simulink model "SwashPlateless_ESC"  (R2025b)
settings: Solver=VariableStepAuto  StartTime=0.0  StopTime=Stop_Time  FixedStep=1e-6  MaxStep=1e-6  RelTol=1e-4
values from neighbouring files (symbols this model uses):
  alpha_bp_rad = deg2rad(alpha_bp_deg)    [Check_alpha_sign.m]    (also in Swash.m)
  alpha_sign = alpha_sign_list(k)    [Check_alpha_sign.m]    (also in Swash.m = 1)
  B = 1.24e-5    (= 1.24e-05)    [Swash.m]
  Imax = 12    [Swash.m]
  J = 1.7e-5    (= 1.7e-05)    [Swash.m]
  Kac = Kic/Kpc    (= 237.676056338)    [Swash.m]
  Kh = 1    [Swash.m]
  Kic = Ra*Wcc    (= 127.23450247)    [Swash.m]
  Kpc = La*Wcc    (= 0.535327388172)    [Swash.m]
  KQ = T0/(W0^2)    (= 3.64756261112e-07)    [Swash.m]
  Kt = 60/(2*pi*KV)    (= 0.0203176523096)    [Swash.m]
  La = 2.84e-4    (= 0.000284)    [Swash.m]
  lambda_f = Kt/(1.5*p)    (= 0.00193501450568)    [Swash.m]
  p = 7    [Swash.m]
  phi_cmd = deg2rad(phi_cmd_deg)    [Check_alpha_sign.m]    (also in Swash.m = deg2rad(30); Sweep_param.m = deg2rad(phi_range_deg(j)))
  rpm_bp = [0 1000 2000 3000 4000 5000 6000]    [Swash.m]
  T0 = 0.10    (= 0.1)    [Swash.m]
  T1 = 0.01    [Check_alpha_sign.m]    (also in Swash.m; Sweep_param.m = T1_range(i))
  tau_h = 0.02    [Swash.m]
  theta_align = deg2rad(-3)    [Swash.m]
  Va_rated = Vdc    (= 22.2)    [Swash.m]
  Vdc = 22.2    [Swash.m]
  Wdisk = 2*pi*fdisk    (= 125.663706144)    [Swash.m]
  Wf = 2*pi*Ff    (= 6283.18530718)    [Swash.m]
undefined symbols (not defined in the file or in its folder): magnitude, plecs
libraries: slpidlib x2, plecslib_extras2 x2, simulink x1
settings Model: Creator=devil  LastModifiedBy=chyuj
settings DebuggingCC: MaxConsecutiveZCsMsg=warning

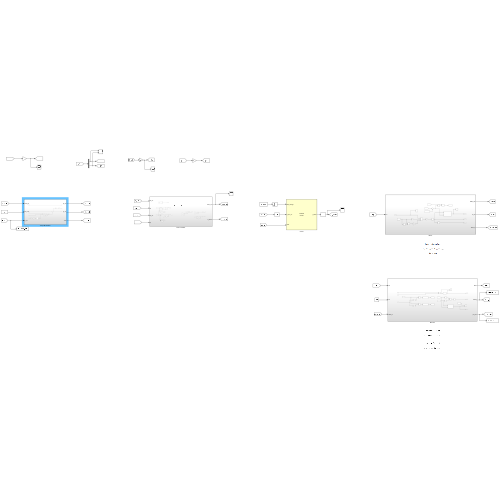
[thumbnail: Simulink's stored preview of the top-level diagram]
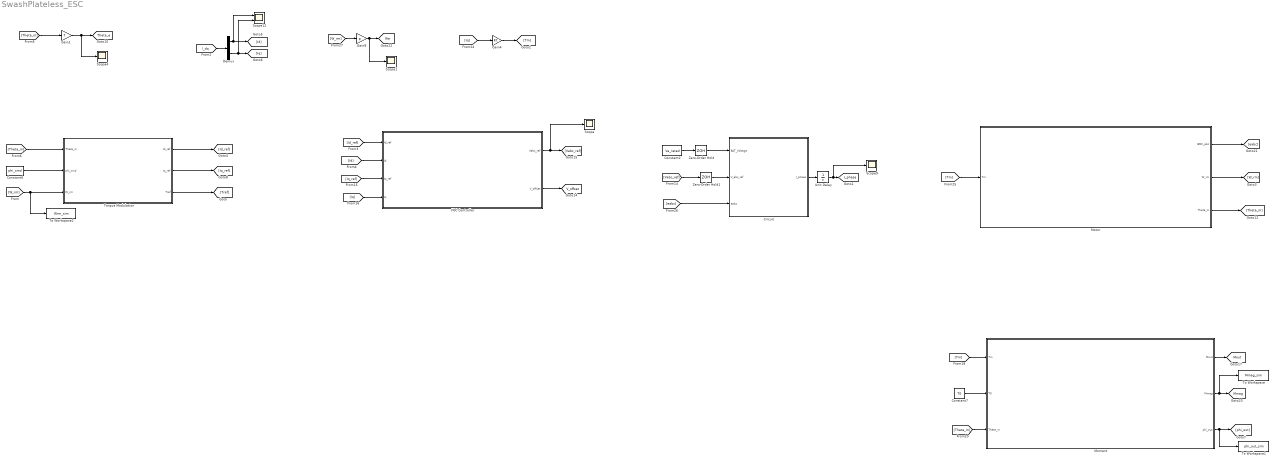
== system SwashPlateless_ESC ==
  Circuit : Subsystem  LoadFcn=plecs('sl', 200);  InitFcn=plecs('sl', 214);  StartFcn=plecs('sl', 208);  StopFcn=plecs('sl', 209);  mask(PlecsCircuit){PLECSData=<binary blob, 6192 chars, not shown>}
      mask prompts: PLECSData "PLECS Data (Do not delete or modify!)"
      mask init:
      | % PLACE CUSTOM INITIALIZATIONS ABOVE
      | % DO NOT REMOVE
      | plecs('sl', 215);
      | % DO NOT REMOVE
      settings: CopyFcn=plecs('sl', 203);  DeleteFcn=plecs('sl', 205);  UndoDeleteFcn=plecs('sl', 206);  PreSaveFcn=plecs('sl', 211);  PostSaveFcn=plecs('sl', 201);  NameChangeFcn=plecs('sl', 210);  DestroyFcn=plecs('sl', 207);  PreCopyFcn=plecs('sl', 216);  OpenFcn=plecs('sl', 202);  ErrorFcn=plerrorfcn
      mask Help: eval('plecs(''help'', ''qthelp:///creatingacircuit.html'')')
      mask Display: disp('PLECS\nCircuit')
  Constant2 : Constant  Value=Va_rated
  Constant6 : Constant  Value=phi_cmd
  Constant7 : Constant  Value=T0
  Demux : Demux  Outputs=2
  FOC Controller : Subsystem
  Gain1 : Gain  Gain=7
  Gain4 : Gain  Gain=Kt
  Gain8 : Gain  Gain=p
  Moment : Subsystem
  Motor : Subsystem
  Scope{,1,4,9} (4 alike) : Scope
      Scope settings: ActiveDisplayYMinimum=-4.6315212670934374  ActiveDisplayYMaximum=5.3776987823320246
      Scope1 settings: ActiveDisplayYMinimum=-1  ActiveDisplayYMaximum=1
      Scope4 settings: ActiveDisplayYMinimum=-1  ActiveDisplayYMaximum=1  DataLoggingVariableName=ScopeData2
      Scope9 settings: ActiveDisplayYMinimum=-6.552499916333363  ActiveDisplayYMaximum=6.5468585971785176  DataLoggingVariableName=ScopeData7
  Scope12 : Scope  NumInputPorts=2
      settings: ActiveDisplayYMinimum=-1.4248324543747475  ActiveDisplayYMaximum=7.121085765539088  DataLoggingVariableName=ScopeData10
  To Workspace : ToWorkspace  VariableName=Mmag_sim  SaveFormat=Timeseries  SampleTime=-1
  To Workspace1 : ToWorkspace  VariableName=phi_out_sim  SaveFormat=Timeseries  SampleTime=-1
  To Workspace2 : ToWorkspace  VariableName=Wrm_sim  SaveFormat=Timeseries  SampleTime=-1
  Torque Modulation : Subsystem
  Unit Delay : UnitDelay  SampleTime=-1  HasFrameUpgradeWarning=on
  Zero-Order Hold : ZeroOrderHold  SampleTime=-1
  Zero-Order Hold1 : ZeroOrderHold  SampleTime=-1
  tag scope: I_phase=global, Mmag=global, Mout=global, Theta_e=global, V_offset=global, We=global
  wires:
  [I_dq] -> Demux/1
  Demux/1 -> Scope12/1, [Id]
  Demux/2 -> Scope12/2, [Iq]
  [Vabc_ref] -> Zero-Order Hold1/1
  Constant2/1 -> Zero-Order Hold/1
  [Theta_m] -> Gain1/1
  Gain1/1 -> Scope4/1, [Theta_e]
  Circuit/1(I_phase) -> Unit Delay/1
  Unit Delay/1 -> Scope9/1, [I_phase]
  Zero-Order Hold/1 -> Circuit/1(BAT_Voltage)
  Zero-Order Hold1/1 -> Circuit/2(V_abc_ref)
  [Iq] -> Gain4/1
  Gain4/1 -> [Tm]
  [eabc] -> Circuit/3(eabc)
  [W_rm] -> Gain8/1
  Gain8/1 -> Scope1/1, [We]
  [Theta_m] -> Torque Modulation/1(Theta_m)
  Constant6/1 -> Torque Modulation/2(phi_cmd)
  Torque Modulation/2(Iq_ref) -> [Iq_ref]
  Torque Modulation/3(Tref) -> [Tref]
  FOC Controller/2(V_offset) -> [V_offset]
  FOC Controller/1(Vabc_ref) -> Scope/1, [Vabc_ref]
  [Id_ref] -> FOC Controller/1(Id_ref)
  [Id] -> FOC Controller/2(Id)
  [Iq_ref] -> FOC Controller/3(Iq_ref)
  [Iq] -> FOC Controller/4(Iq)
  [Tm] -> Moment/1(Tm)
  Constant7/1 -> Moment/2(T0)
  [Theta_m] -> Moment/3(Theta_m)
  Moment/1(Mout) -> [Mout]
  [Tm] -> Motor/1(Tm)
  Motor/1(BMF_abc) -> [eabc]
  Motor/2(W_rm) -> [W_rm]
  Motor/3(Theta_m) -> [Theta_m]
  Torque Modulation/1(Id_ref) -> [Id_ref]
  Moment/2(Mmag) -> To Workspace/1, [Mmag]
  Moment/3(phi_out) -> To Workspace1/1, [phi_out]
  [W_rm] -> To Workspace2/1, Torque Modulation/3(W_rm)

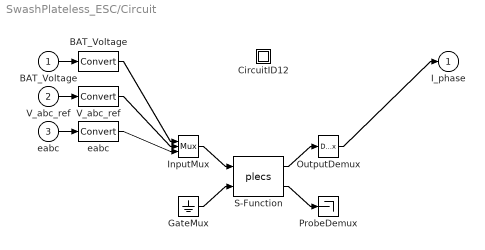
== system SwashPlateless_ESC/Circuit ==
  BAT_Voltage : Inport  PortDimensions=1
  V_abc_ref : Inport  Port=2  PortDimensions=3
  eabc : Inport  Port=3  PortDimensions=3
  " BAT_Voltage " : DataTypeConversion
  " CircuitID12 " : Subsystem
  " GateMux " : Ground
  " InputMux " : Mux  Inputs=[ 1 3 3 ]
  " OutputDemux " : Demux  Outputs=[ 3 ]
  " ProbeDemux " : Terminator
  " S-Function " : S-Function  FunctionName=plecs  SFunctionDeploymentMode=off  EnableBusSupport=off
  " V_abc_ref " : DataTypeConversion
  " eabc " : DataTypeConversion
  I_phase : Outport  PortDimensions=3
  wires:
  " InputMux "/1 -> " S-Function "/1
  " GateMux "/1 -> " S-Function "/2
  " S-Function "/1 -> " OutputDemux "/1
  " S-Function "/2 -> " ProbeDemux "/1
  BAT_Voltage/1 -> " BAT_Voltage "/1
  " BAT_Voltage "/1 -> " InputMux "/1
  V_abc_ref/1 -> " V_abc_ref "/1
  " V_abc_ref "/1 -> " InputMux "/2
  eabc/1 -> " eabc "/1
  " eabc "/1 -> " InputMux "/3
  " OutputDemux "/1 -> I_phase/1

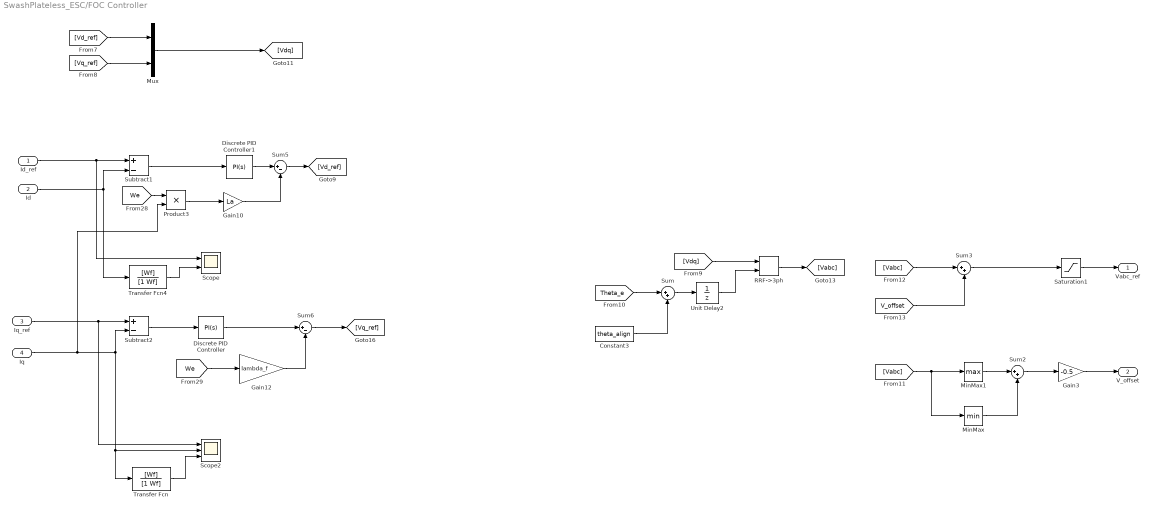
== system SwashPlateless_ESC/FOC Controller ==
  Id_ref : Inport
  Id : Inport  Port=2
  Iq_ref : Inport  Port=3
  Iq : Inport  Port=4
  Constant3 : Constant  Value=theta_align
  Discrete PID Controller : slpidlib/PID Controller  Controller=PI  Form=Parallel  TimeDomain=Continuous-time  UseExternalTs=off  SampleTime=-1  IntegratorMethod=Forward Euler  FilterMethod=Forward Euler  ControllerParametersSource=internal  P=Kpc  I=Kic  UseKiTs=off  D=0  UseExternalDerivativeSource=off  N=100  UseFilter=on  TunerSelectOption=Transfer Function Based (PID Tuner App)  InitialConditionSource=internal  InitialConditionForIntegrator=0  InitialConditionForFilter=0  DifferentiatorICPrevScaledInput=0  ExternalReset=none  TrackingMode=off  Kt=1  LimitOutput=on  SatLimitsSource=internal  UpperSaturationLimit=Vdc/sqrt(3)  LowerSaturationLimit=-Vdc/sqrt(3)  LinearizeAsGain=on  AntiWindupMode=back-calculation  Kb=Kac  LimitIntegrator=off  UpperIntegratorSaturationLimit=inf  LowerIntegratorSaturationLimit=-inf  POutMin=[]  POutMax=[]  IOutMin=[]  IOutMax=[]  DOutMin=[]  DOutMax=[]  NOutMin=[]  NOutMax=[]  SumOutMin=[]  SumOutMax=[]  SaturationOutMin=[]  SaturationOutMax=[]  PParamMin=[]  PParamMax=[]  IParamMin=[]  IParamMax=[]  DParamMin=[]  DParamMax=[]  NParamMin=[]  NParamMax=[]  KbParamMin=[]  KbParamMax=[]  KtParamMin=[]  KtParamMax=[]  KbOutMin=[]  KbOutMax=[]  KtOutMin=[]  KtOutMax=[]  IntegratorOutMin=[]  IntegratorOutMax=[]  FilterOutMin=[]  FilterOutMax=[]  SumI1OutMin=[]  SumI1OutMax=[]  SumI2OutMin=[]  SumI2OutMax=[]  SumI3OutMin=[]  SumI3OutMax=[]  SumI4OutMin=[]  SumI4OutMax=[]  SumDOutMin=[]  SumDOutMax=[]  DifferentiatorOutMin=[]  DifferentiatorOutMax=[]  FilterDiffOutCoefMin=[]  FilterDiffOutCoefMax=[]  ReciprocalOutMin=[]  ReciprocalOutMax=[]  SumDenOutMin=[]  SumDenOutMax=[]  SumNumOutMin=[]  SumNumOutMax=[]  DivideOutMin=[]  DivideOutMax=[]  UdiffTsProdOutMin=[]  UdiffTsProdOutMax=[]  NTsProdOutMin=[]  NTsProdOutMax=[]  UintegralTsProdOutMin=[]  UintegralTsProdOutMax=[]  UngainTsProdOutMin=[]  UngainTsProdOutMax=[]  ClampingZeroOutDataTypeStr=Inherit: Inherit via back propagation  ClampingZeroOutMin=[]  ClampingZeroOutMax=[]  FilterDenConstantOutDataTypeStr=Inherit: Inherit via back propagation  FilterDenConstantOutMin=[]  FilterDenConstantOutMax=[]  PCopyOutDataTypeStr=Inherit: Inherit via back propagation  PCopyOutMin=[]  PCopyOutMax=[]  NCopyOutDataTypeStr=Inherit: Inherit via back propagation  NCopyOutMin=[]  NCopyOutMax=[]  IntegratorContinuousStateAttributes=''  IntegratorStateMustResolveToSignalObject=off  IntegratorRTWStateStorageClass=Auto  FilterContinuousStateAttributes=''  FilterStateMustResolveToSignalObject=off  FilterRTWStateStorageClass=Auto  ParallelPVariant=InternalParameters  IdealPVariant=Disabled  IVariant=InternalParameters  DVariant=Disabled  IntegratorVariant=Continuous  SatVariant=Enabled  AWVariant=BackCalculation  PCopyVariant=Disabled  TRVariant=Disabled  FdbkBlocksVariant=Forward  IdealPFdbkVariant=Disabled  SatFdbkVariant=Disabled  DerivativeFilterVariant=Disabled  NVariant=Disabled  NCopyVariant=Disabled_SignalSpec  FilterICVariant=Disabled  IntegratorICVariant=InternalICs  ExternalResetVariant=Disabled  TRSumVariant=Passthrough  SumFdbkVariant=Disabled  SumVariant=Sum_PI  TsampFilterVariant=InternalTs  TsampNgainVariant=Passthrough  TsampIntegralVariant=Disabled_SignalSpec  ExternalSaturationOutDataTypeStr=Inherit: Same as second input  DerivativeSourceVariant=Disabled  PreIntVariant=InternalPreInt
      settings: LibrarySourceBlock=simulink/Discrete/Discrete PID Controller
  Discrete PID Controller1 : slpidlib/PID Controller  Controller=PI  Form=Parallel  TimeDomain=Continuous-time  UseExternalTs=off  SampleTime=-1  IntegratorMethod=Forward Euler  FilterMethod=Forward Euler  ControllerParametersSource=internal  P=Kpc  I=Kic  UseKiTs=off  D=0  UseExternalDerivativeSource=off  N=100  UseFilter=on  TunerSelectOption=Transfer Function Based (PID Tuner App)  InitialConditionSource=internal  InitialConditionForIntegrator=0  InitialConditionForFilter=0  DifferentiatorICPrevScaledInput=0  ExternalReset=none  TrackingMode=off  Kt=1  LimitOutput=on  SatLimitsSource=internal  UpperSaturationLimit=Vdc/sqrt(3)  LowerSaturationLimit=-Vdc/sqrt(3)  LinearizeAsGain=on  AntiWindupMode=back-calculation  Kb=Kac  LimitIntegrator=off  UpperIntegratorSaturationLimit=inf  LowerIntegratorSaturationLimit=-inf  POutMin=[]  POutMax=[]  IOutMin=[]  IOutMax=[]  DOutMin=[]  DOutMax=[]  NOutMin=[]  NOutMax=[]  SumOutMin=[]  SumOutMax=[]  SaturationOutMin=[]  SaturationOutMax=[]  PParamMin=[]  PParamMax=[]  IParamMin=[]  IParamMax=[]  DParamMin=[]  DParamMax=[]  NParamMin=[]  NParamMax=[]  KbParamMin=[]  KbParamMax=[]  KtParamMin=[]  KtParamMax=[]  KbOutMin=[]  KbOutMax=[]  KtOutMin=[]  KtOutMax=[]  IntegratorOutMin=[]  IntegratorOutMax=[]  FilterOutMin=[]  FilterOutMax=[]  SumI1OutMin=[]  SumI1OutMax=[]  SumI2OutMin=[]  SumI2OutMax=[]  SumI3OutMin=[]  SumI3OutMax=[]  SumI4OutMin=[]  SumI4OutMax=[]  SumDOutMin=[]  SumDOutMax=[]  DifferentiatorOutMin=[]  DifferentiatorOutMax=[]  FilterDiffOutCoefMin=[]  FilterDiffOutCoefMax=[]  ReciprocalOutMin=[]  ReciprocalOutMax=[]  SumDenOutMin=[]  SumDenOutMax=[]  SumNumOutMin=[]  SumNumOutMax=[]  DivideOutMin=[]  DivideOutMax=[]  UdiffTsProdOutMin=[]  UdiffTsProdOutMax=[]  NTsProdOutMin=[]  NTsProdOutMax=[]  UintegralTsProdOutMin=[]  UintegralTsProdOutMax=[]  UngainTsProdOutMin=[]  UngainTsProdOutMax=[]  ClampingZeroOutDataTypeStr=Inherit: Inherit via back propagation  ClampingZeroOutMin=[]  ClampingZeroOutMax=[]  FilterDenConstantOutDataTypeStr=Inherit: Inherit via back propagation  FilterDenConstantOutMin=[]  FilterDenConstantOutMax=[]  PCopyOutDataTypeStr=Inherit: Inherit via back propagation  PCopyOutMin=[]  PCopyOutMax=[]  NCopyOutDataTypeStr=Inherit: Inherit via back propagation  NCopyOutMin=[]  NCopyOutMax=[]  IntegratorContinuousStateAttributes=''  IntegratorStateMustResolveToSignalObject=off  IntegratorRTWStateStorageClass=Auto  FilterContinuousStateAttributes=''  FilterStateMustResolveToSignalObject=off  FilterRTWStateStorageClass=Auto  ParallelPVariant=InternalParameters  IdealPVariant=Disabled  IVariant=InternalParameters  DVariant=Disabled  IntegratorVariant=Continuous  SatVariant=Enabled  AWVariant=BackCalculation  PCopyVariant=Disabled  TRVariant=Disabled  FdbkBlocksVariant=Forward  IdealPFdbkVariant=Disabled  SatFdbkVariant=Disabled  DerivativeFilterVariant=Disabled  NVariant=Disabled  NCopyVariant=Disabled_SignalSpec  FilterICVariant=Disabled  IntegratorICVariant=InternalICs  ExternalResetVariant=Disabled  TRSumVariant=Passthrough  SumFdbkVariant=Disabled  SumVariant=Sum_PI  TsampFilterVariant=InternalTs  TsampNgainVariant=Passthrough  TsampIntegralVariant=Disabled_SignalSpec  ExternalSaturationOutDataTypeStr=Inherit: Same as second input  DerivativeSourceVariant=Disabled  PreIntVariant=InternalPreInt
      settings: LibrarySourceBlock=simulink/Discrete/Discrete PID Controller
  Gain10 : Gain  Gain=La
  Gain12 : Gain  Gain=lambda_f
  Gain3 : Gain  Gain=-0.5
  MinMax : MinMax
  MinMax1 : MinMax  Function=max
  Mux : Mux  Inputs=2
  Product3 : Product
  RRF->3ph : plecslib_extras2/Transformations/RRF->3ph
      settings: SourceProductName=PLECS Extras
  Saturation1 : Saturate  UpperLimit=0.49*Vdc  LowerLimit=-0.49*Vdc
  Scope : Scope  NumInputPorts=2
      settings: ActiveDisplayYMinimum=-2.7389602608191588  ActiveDisplayYMaximum=3.7222976897141629
  Scope2 : Scope  NumInputPorts=3
      settings: ActiveDisplayYMinimum=4.9459750721392517  ActiveDisplayYMaximum=5.2413041360162866  DataLoggingVariableName=ScopeData2
  Subtract1 : Sum  Inputs=+-
  Subtract2 : Sum  Inputs=+-
  Sum : Sum  Inputs=|++
  Sum2 : Sum  Inputs=|++
  Sum3 : Sum  Inputs=|++
  Sum5 : Sum  Inputs=|+-
  Sum6 : Sum  Inputs=|+-
  Transfer Fcn : TransferFcn  Numerator=[Wf]  Denominator=[1 Wf]
  Transfer Fcn4 : TransferFcn  Numerator=[Wf]  Denominator=[1 Wf]
  Unit Delay2 : UnitDelay  SampleTime=-1  HasFrameUpgradeWarning=on
  Vabc_ref : Outport
  V_offset : Outport  Port=2
  wires:
  Sum5/1 -> [Vd_ref]
  [Vdq] -> RRF->3ph/1
  Id_ref/1 -> Scope/1, Subtract1/1
  Iq/1 -> Product3/2, Subtract2/2, Transfer Fcn/1, Scope2/2
  Id/1 -> Transfer Fcn4/1, Subtract1/2
  Sum6/1 -> [Vq_ref]
  Iq_ref/1 -> Scope2/1, Subtract2/1
  Discrete PID Controller1/1 -> Sum5/1
  MinMax/1 -> Sum2/2
  Subtract2/1 -> Discrete PID Controller/1
  Constant3/1 -> Sum/2
  Mux/1 -> [Vdq]
  [Theta_e] -> Sum/1
  [Vabc] -> MinMax/1, MinMax1/1
  Gain10/1 -> Sum5/2
  [V_offset] -> Sum3/2
  Subtract1/1 -> Discrete PID Controller1/1
  [Vd_ref] -> Mux/1
  Transfer Fcn/1 -> Scope2/3
  Discrete PID Controller/1 -> Sum6/1
  Gain12/1 -> Sum6/2
  Sum2/1 -> Gain3/1
  Transfer Fcn4/1 -> Scope/2
  [We] -> Product3/1
  Unit Delay2/1 -> RRF->3ph/2
  Sum/1 -> Unit Delay2/1
  [Vq_ref] -> Mux/2
  [Vabc] -> Sum3/1
  Sum3/1 -> Saturation1/1
  [We] -> Gain12/1
  Gain3/1 -> V_offset/1
  Product3/1 -> Gain10/1
  MinMax1/1 -> Sum2/1
  RRF->3ph/1 -> [Vabc]
  Saturation1/1 -> Vabc_ref/1

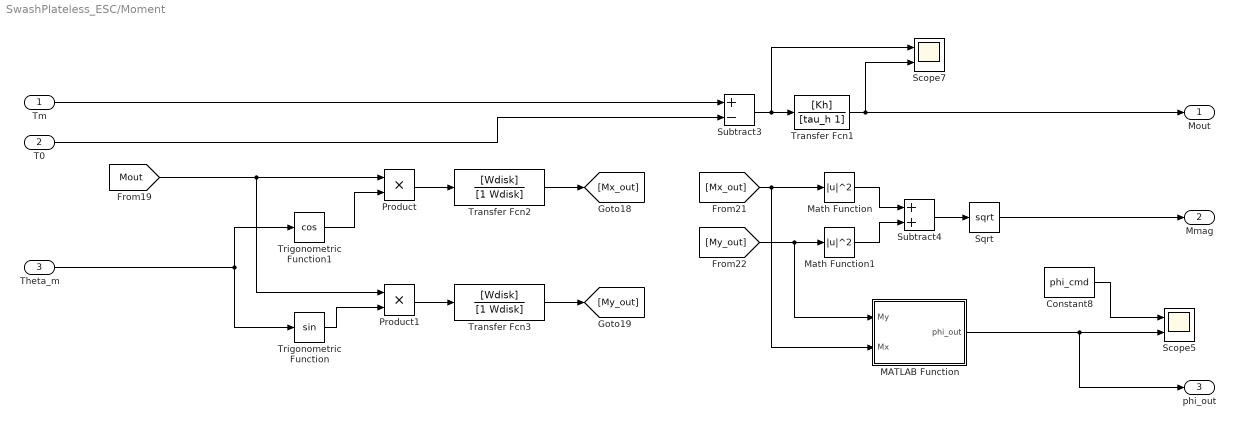
== system SwashPlateless_ESC/Moment ==
  Tm : Inport
  T0 : Inport  Port=2
  Theta_m : Inport  Port=3
  Constant8 : Constant  Value=phi_cmd
  MATLAB Function : MATLAB Function  TreatAsAtomicUnit=on
  Math Function : Math  Operator=magnitude^2
  Math Function1 : Math  Operator=magnitude^2
  Product : Product
  Product1 : Product
  Scope5 : Scope  NumInputPorts=2
      settings: ActiveDisplayYMinimum=-1  ActiveDisplayYMaximum=1  DataLoggingVariableName=ScopeData3
  Scope7 : Scope  NumInputPorts=2
      settings: ActiveDisplayYMinimum=-0.11471706424926205  ActiveDisplayYMaximum=0.032453578243358414  DataLoggingVariableName=ScopeData5
  Sqrt : Sqrt
  Subtract3 : Sum  Inputs=+-
  Subtract4 : Sum
  Transfer Fcn1 : TransferFcn  Numerator=[Kh]  Denominator=[tau_h 1]
  Transfer Fcn2 : TransferFcn  Numerator=[Wdisk]  Denominator=[1 Wdisk]
  Transfer Fcn3 : TransferFcn  Numerator=[Wdisk]  Denominator=[1 Wdisk]
  Trigonometric Function : Trigonometry
  Trigonometric Function1 : Trigonometry  Operator=cos
  Mout : Outport
  Mmag : Outport  Port=2
  phi_out : Outport  Port=3
  wires:
  Math Function1/1 -> Subtract4/2
  Theta_m/1 -> Trigonometric Function/1, Trigonometric Function1/1
  [Mx_out] -> MATLAB Function/2(Mx), Math Function/1
  Transfer Fcn2/1 -> [Mx_out]
  MATLAB Function/1(phi_out) -> phi_out/1, Scope5/2
  Product/1 -> Transfer Fcn2/1
  Constant8/1 -> Scope5/1
  Transfer Fcn1/1 -> Mout/1, Scope7/2
  Product1/1 -> Transfer Fcn3/1
  Subtract3/1 -> Scope7/1, Transfer Fcn1/1
  [My_out] -> MATLAB Function/1(My), Math Function1/1
  Transfer Fcn3/1 -> [My_out]
  [Mout] -> Product1/1, Product/1
  Trigonometric Function1/1 -> Product/2
  Subtract4/1 -> Sqrt/1
  Math Function/1 -> Subtract4/1
  Trigonometric Function/1 -> Product1/2
  T0/1 -> Subtract3/2
  Tm/1 -> Subtract3/1
  Sqrt/1 -> Mmag/1

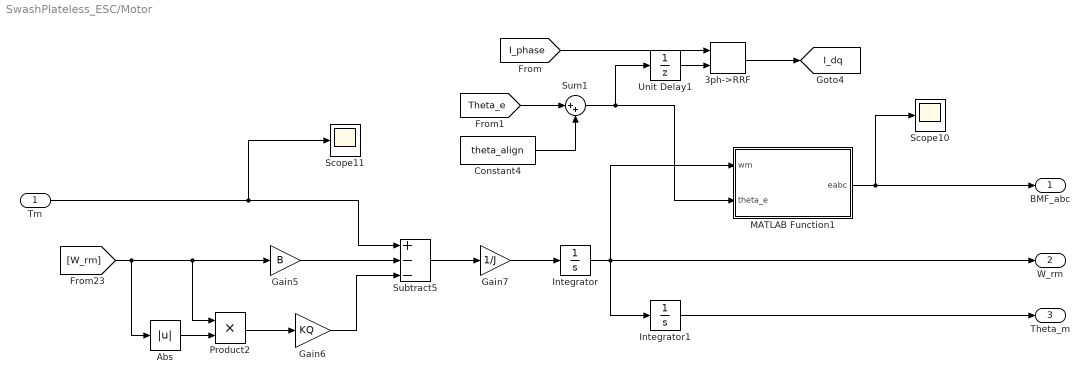
== system SwashPlateless_ESC/Motor ==
  Tm : Inport
  3ph->RRF : plecslib_extras2/Transformations/3ph->RRF
      settings: SourceProductName=PLECS Extras
  Abs : Abs  SaturateOnIntegerOverflow=off
  Constant4 : Constant  Value=theta_align
  Gain5 : Gain  Gain=B
  Gain6 : Gain  Gain=KQ
  Gain7 : Gain  Gain=1/J
  Integrator : Integrator
  Integrator1 : Integrator
  MATLAB Function1 : MATLAB Function  TreatAsAtomicUnit=on
  Product2 : Product
  Scope10 : Scope
      settings: ActiveDisplayYMinimum=-1  ActiveDisplayYMaximum=1  DataLoggingVariableName=ScopeData8
  Scope11 : Scope
      settings: ActiveDisplayYMinimum=-0.44393553229657284  ActiveDisplayYMaximum=0.21891341323034258  DataLoggingVariableName=ScopeData9
  Subtract5 : Sum  Inputs=+--
  Sum1 : Sum  Inputs=|++
  Unit Delay1 : UnitDelay  SampleTime=-1  HasFrameUpgradeWarning=on
  BMF_abc : Outport
  W_rm : Outport  Port=2
  Theta_m : Outport  Port=3
  tag scope: I_dq=global
  wires:
  Integrator/1 -> W_rm/1, MATLAB Function1/1(wm), Integrator1/1
  Sum1/1 -> MATLAB Function1/2(theta_e), Unit Delay1/1
  [Theta_e] -> Sum1/1
  Gain7/1 -> Integrator/1
  MATLAB Function1/1(eabc) -> BMF_abc/1, Scope10/1
  Integrator1/1 -> Theta_m/1
  [I_phase] -> 3ph->RRF/1
  Tm/1 -> Scope11/1, Subtract5/1
  Subtract5/1 -> Gain7/1
  Unit Delay1/1 -> 3ph->RRF/2
  Product2/1 -> Gain6/1
  Constant4/1 -> Sum1/2
  Gain6/1 -> Subtract5/3
  Gain5/1 -> Subtract5/2
  Abs/1 -> Product2/2
  3ph->RRF/1 -> [I_dq]
  [W_rm] -> Abs/1, Product2/1, Gain5/1

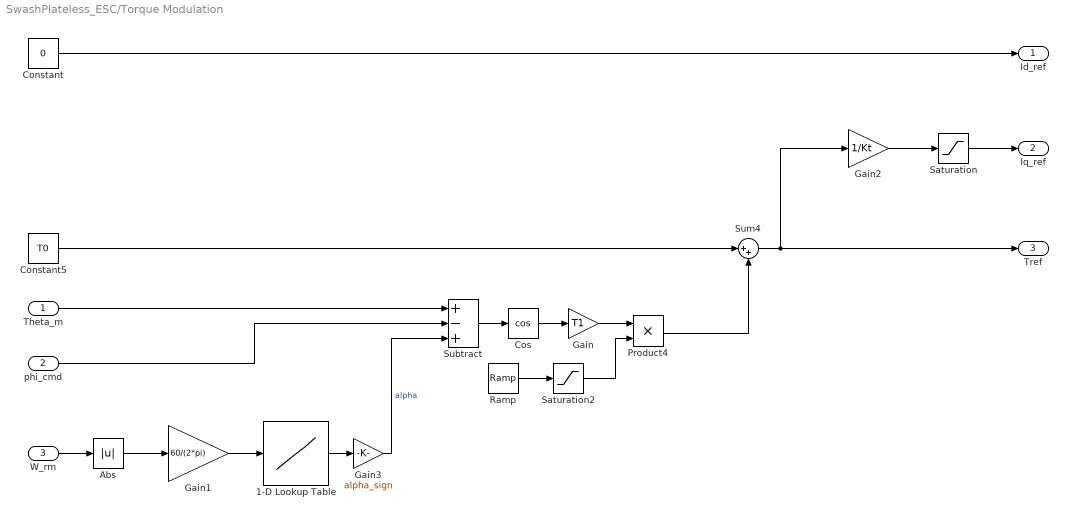
== system SwashPlateless_ESC/Torque Modulation ==
  Theta_m : Inport
  phi_cmd : Inport  Port=2
  W_rm : Inport  Port=3
  1-D Lookup Table : Lookup_n-D  NumberOfTableDimensions=1  BreakpointsForDimension1=rpm_bp  Table=alpha_bp_rad  InternalRulePriority=Speed  RndMeth=Simplest
  Abs : Abs  SaturateOnIntegerOverflow=off
  Constant : Constant  Value=0
  Constant5 : Constant  Value=T0
  Cos : Trigonometry  Operator=cos
  Gain : Gain  Gain=T1
  Gain1 : Gain  Gain=60/(2*pi)
  Gain2 : Gain  Gain=1/Kt
  Gain3 : Gain  Gain=alpha_sign
  Product4 : Product
  Ramp : simulink/Sources/Ramp  slope=50  start=0.02  InitialOutput=0
  Saturation : Saturate  UpperLimit=Imax  LowerLimit=-Imax
  Saturation2 : Saturate  UpperLimit=1  LowerLimit=0
  Subtract : Sum  Inputs=+-+
  Sum4 : Sum  Inputs=|++
  Id_ref : Outport
  Iq_ref : Outport  Port=2
  Tref : Outport  Port=3
  wires:
  Saturation2/1 -> Product4/2
  Product4/1 -> Sum4/2
  Gain/1 -> Product4/1
  Cos/1 -> Gain/1
  Constant5/1 -> Sum4/1
  Subtract/1 -> Cos/1
  Ramp/1 -> Saturation2/1
  Gain2/1 -> Saturation/1
  Saturation/1 -> Iq_ref/1
  phi_cmd/1 -> Subtract/2
  Theta_m/1 -> Subtract/1
  Sum4/1 -> Gain2/1, Tref/1
  Constant/1 -> Id_ref/1
  W_rm/1 -> Abs/1
  Abs/1 -> Gain1/1
  Gain1/1 -> 1-D Lookup Table/1
  1-D Lookup Table/1 -> Gain3/1
  Gain3/1 -> Subtract/3  "alpha"

== system SwashPlateless_ESC/Circuit/ CircuitID12  ==

== matlab function SwashPlateless_ESC/Moment/MATLAB Function ==
  data: My input; phi_out output; Mx input
function phi_out = fcn(My, Mx)
phi_out = atan2(My, Mx);
end

== matlab function SwashPlateless_ESC/Motor/MATLAB Function1 ==
  data: wm input; eabc output; theta_e input
function eabc = bemf_abc(wm, theta_e)
% MN3110 KV470 sinusoidal back-EMF model

KV = 470;
p = 7;

Kt = 60/(2*pi*KV);
lambda_f = Kt/(1.5*p);

we = p*wm;

ea = we*lambda_f*sin(theta_e);
eb = we*lambda_f*sin(theta_e - 2*pi/3);
ec = we*lambda_f*sin(theta_e + 2*pi/3);

eabc = [ea; eb; ec];
end
